simulink model "Rocket_PD_Controller"  (R2025a)
settings: Solver=VariableStepAuto  StartTime=0.0  StopTime=10.0  RelTol=1e-3
settings Model: Creator=pepem  LastModifiedBy=pepem

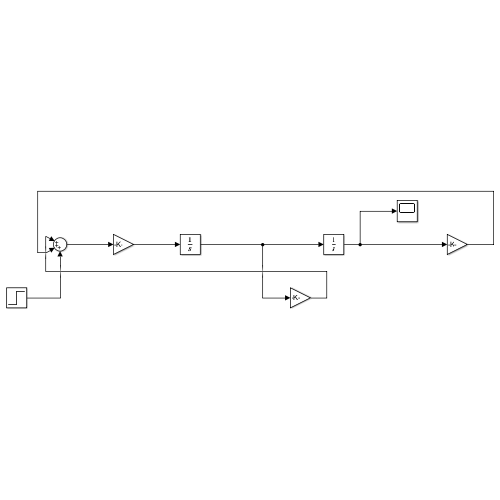
[thumbnail: Simulink's stored preview of the top-level diagram]
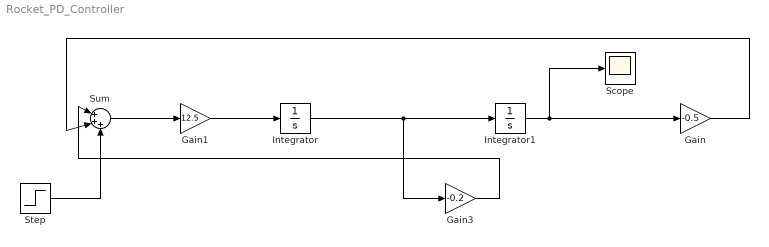
== system Rocket_PD_Controller ==
  Gain : Gain  Gain=-0.5
  Gain1 : Gain  Gain=12.5
  Gain3 : Gain  Gain=-0.2
  Integrator : Integrator
  Integrator1 : Integrator
  Scope : Scope
      settings: ActiveDisplayYMinimum=-1  ActiveDisplayYMaximum=1
  Step : Step  SampleTime=0
  Sum : Sum  Inputs=|+++
  wires:
  Gain1/1 -> Integrator/1
  Sum/1 -> Gain1/1
  Integrator1/1 -> Scope/1, Gain/1
  Integrator/1 -> Gain3/1, Integrator1/1
  Gain3/1 -> Sum/1
  Gain/1 -> Sum/2
  Step/1 -> Sum/3
